simulink model "DDCU_wxt_v02_forA"  (R2014a)
settings: Solver=FixedStepDiscrete  StartTime=0.0  StopTime=50  FixedStep=0.0005  RelTol=1e-3
InitFcn:
  | Veh_Par_wxt
values from neighbouring files (symbols this model uses):
  ag_thr = 0.4*g    (= 3.924)    [Veh_Par_wxt.m]
  B = 2.25    [Veh_Par_wxt.m]
  bra_pre_em = 12    [Veh_Par_wxt.m]
  bra_pre_gz2 = 12/3    (= 4)    [Veh_Par_wxt.m]
  bra_pre_gz34 = 12/3    (= 4)    [Veh_Par_wxt.m]
  bra_pre_yd = 12/2    (= 6)    [Veh_Par_wxt.m]
  brakepre_dem_data = [0 1 2 3 4 5 6 7 8 9 10 11 12]    [Veh_Par_wxt.m]
  brakeTrq_dem_data = [0 218.198 436.396 654.594 872.792 1090.99 1309.188 1527.386 1745.584 1963.782 2181.98 2400.178 2618.376]    [Veh_Par_wxt.m]
  bratrq_max = 4*2618.376    (= 10473.504)    [Veh_Par_wxt.m]
  eff_tran = 0.75    [Veh_Par_wxt.m]
  G = Mass*g    (= 36297)    [Veh_Par_wxt.m]
  kd1 = 1    [Veh_Par_wxt.m]
  kd2 = 1    [Veh_Par_wxt.m]
  kd3 = 1    [Veh_Par_wxt.m]
  ki1 = 1    [Veh_Par_wxt.m]
  ki2 = 1    [Veh_Par_wxt.m]
  ki3 = 1    [Veh_Par_wxt.m]
  kp1 = 1    [Veh_Par_wxt.m]
  kp2 = 1    [Veh_Par_wxt.m]
  kp3 = 1    [Veh_Par_wxt.m]
  L = 3.12    [Veh_Par_wxt.m]
  Radius = 0.20    (= 0.2)    [Veh_Par_wxt.m]
  s_opt_yi_add = 0.05    [Veh_Par_wxt.m]
  s_opt_zhuan_add = 0.05    [Veh_Par_wxt.m]
  spd_map_mot = [0 100 200 300 360 400 500 600 700 800 900]*tras_ratio    [Veh_Par_wxt.m]
  speed_thr_park = 5/3.6/Radius*30/pi    (= 66.3145596216)    [Veh_Par_wxt.m]
  trq_map_mot = [1200 1200 1200 1200 1200 1080 864 720 617 540 480]/tras_ratio    [Veh_Par_wxt.m]
  v_thr1_b = 5    [Veh_Par_wxt.m]
  v_thr2_b = 20    [Veh_Par_wxt.m]
  v_thr_park = 5    [Veh_Par_wxt.m]
undefined symbols (not defined in the file or in its folder): DiscIntNeverNeededParam
libraries: simulink x201, ec5744lib x19
(part 1 of 9)
settings Model: Creator=wxt  LastModifiedBy=wxt
settings OptimizationCC: InlineParams=on  InlineInvariantSignals=on  ExpressionFolding=off  RollThreshold=9  StateBitsets=on  DataBitsets=on  UseTempVars=on  ZeroExternalMemoryAtStartup=off  ZeroInternalMemoryAtStartup=off  EfficientFloat2IntCast=on  OptimizeModelRefInitCode=on  LifeSpan=1
settings DebuggingCC: InheritedTsInSrcMsg=none
settings HardwareCC: ProdLargestAtomicInteger=Long  ProdLargestAtomicFloat=Double  ProdIntDivRoundTo=Zero  ProdEndianess=BigEndian  ProdHWDeviceType=Freescale MPC5500
settings RTWCC: SystemTargetFile=ec5744.tlc  MakeCommand=make_rtw optimized_fixed_point=1  GenerateMakefile=off  TemplateMakefile=ec5744_lcc.tmf  PostCodeGenCommand=ec5744_pst_s2(buildInfo)  Description=Target for EC5744  GenerateReport=on  ProcessScript=ec5744_make_rtw_hook  IncludeHyperlinkInReport=on  LaunchReport=on
settings CodeAppCC: IgnoreCustomStorageClasses=off
settings STFCustomTargetCC: ModelReferenceCompliant=off  ConcurrentExecutionCompliant=off  IncludeMdlTerminateFcn=off  GeneratePreprocessorConditionals=Use local settings  CombineOutputUpdateFcns=on  SuppressErrorStatus=on  ERTCustomFileBanners=on  SupportContinuousTime=off  SupportNonInlinedSFcns=off  MATLABClassNameForMDSCustomization=Simulink.SoftwareTarget.ERTCustomization  GRTInterface=off  SystemTargetFile=ec5744.tlc
settings ERTTargetCC: GenerateSampleERTMain=off  ModelReferenceCompliant=off  IncludeMdlTerminateFcn=off  SuppressErrorStatus=on  GenerateASAP2=on  ERTSrcFileBannerTemplate=ec5744_code_template.cgt  ERTHdrFileBannerTemplate=ec5744_code_template.cgt  ERTDataSrcFileTemplate=ec5744_code_template.cgt  ERTDataHdrFileTemplate=ec5744_code_template.cgt  ERTCustomFileTemplate=ec5744_file_process.tlc

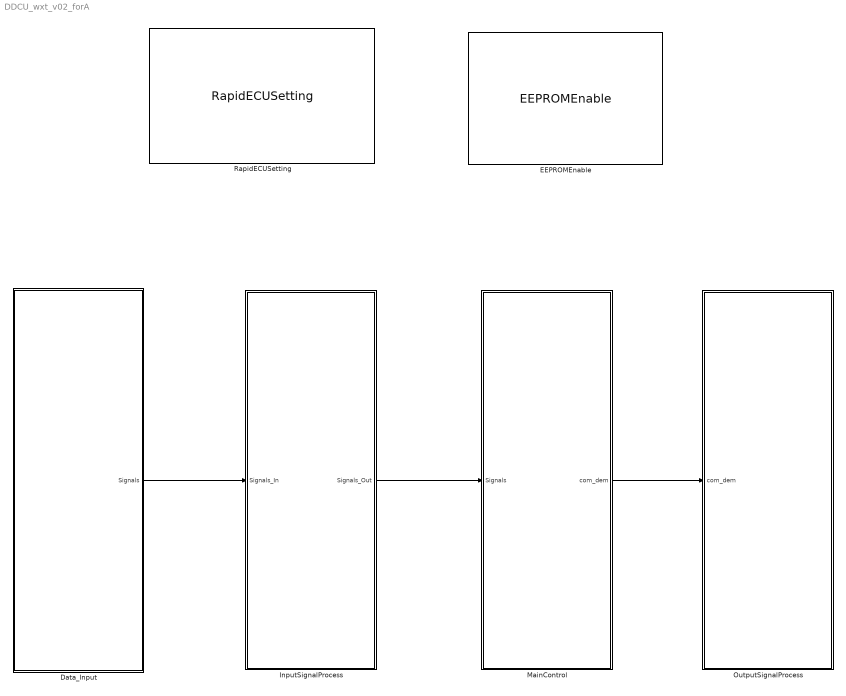
== system DDCU_wxt_v02_forA ==
  Data_Input : Subsystem
  EEPROMEnable : ec5744lib/RapidECU_U3/09MemoryManagement/EEPROMEnable  eepromenable=on
  InputSignalProcess : Subsystem
  MainControl : Subsystem
  OutputSignalProcess : Subsystem
  RapidECUSetting : ec5744lib/RapidECU_U3/RapidECUSetting
      link override CAN: apdf=4  bpdf=4  cpdf=4  acmt=Extended(29-bit ID)  bcmt=Extended(29-bit ID)
      link override LIN: abrt=19200
  wires:
  Data_Input/1(Signals) -> InputSignalProcess/1(Signals_In)
  InputSignalProcess/1(Signals_Out) -> MainControl/1(Signals)
  MainControl/1(com_dem) -> OutputSignalProcess/1(com_dem)

== system DDCU_wxt_v02_forA/Data_Input ==
  Battery : Subsystem
  BraSystem : Subsystem
  Bus Creator : BusCreator  Inputs=6
  DriveMotor : Subsystem
  ESC2VCU : Subsystem
  Ground : Ground
  Ground1 : Ground
  Ground2 : Ground
  HCU2VCU : Subsystem
  IMU : Subsystem
  MCU2VCU : Subsystem
  Subsystem : Subsystem
  Suspension : Subsystem
  YaoKong : Subsystem
  Signals : Outport
  wires:
  DriveMotor/1(DriveMotor) -> Bus Creator/2
  BraSystem/1(BraPre) -> Bus Creator/3
  YaoKong/1(YaoKong_dem) -> Bus Creator/1
  IMU/1(IMU) -> Bus Creator/4
  Suspension/1(Center_of_Mass) -> Bus Creator/5
  Bus Creator/1 -> Signals/1
  Battery/1(Bat) -> Bus Creator/6
  Ground/1 -> Suspension/1(location_center)
  Ground2/1 -> Battery/2(pwr_chg_bat)
  Ground1/1 -> Battery/1(pwr_dis_bat)
  HCU2VCU/5(Turn_Out) -> YaoKong/3(steer_dem)
  HCU2VCU/6(AccBra_Out) -> YaoKong/2(acc_dem)
  HCU2VCU/7(Mode2_Out) -> Subsystem/1(Mode2_Out)
  HCU2VCU/8(Mode1_Out) -> Subsystem/2(Mode1_Out)
  Subsystem/1(mode_dem) -> YaoKong/1(mode_dem)
  MCU2VCU/2(M1Speed_Out) -> DriveMotor/1(speed_act_lf)
  MCU2VCU/7(M1Torque_Out) -> DriveMotor/2(trq_act_lf)
  MCU2VCU/8(M1FaultGrade_Out) -> DriveMotor/5(guzhang_lf)
  MCU2VCU/10(M1TqLimit_Out) -> DriveMotor/3(trqlimU_dig_lf)
  MCU2VCU/14(M3Speed_Out) -> DriveMotor/6(speed_act_lr)
  MCU2VCU/19(M3Torque_Out) -> DriveMotor/7(trq_act_lr)
  MCU2VCU/21(M3FaultGrade_Out) -> DriveMotor/10(guzhang_lr)
  MCU2VCU/22(M3TqLimit_Out) -> DriveMotor/8(trqlimU_dig_lr)
  MCU2VCU/25(M2Torque_Out) -> DriveMotor/12(trq_act_rf)
  MCU2VCU/27(M2Speed_Out) -> DriveMotor/11(speed_act_rf)
  MCU2VCU/33(M2FaultGrade_Out) -> DriveMotor/15(guzhang_rf)
  MCU2VCU/34(M2TqLimit_Out) -> DriveMotor/13(trqlimU_dig_rf)
  MCU2VCU/38(M4Speed_Out) -> DriveMotor/16(speed_act_rr)
  MCU2VCU/43(M4Torque_Out) -> DriveMotor/17(trq_act_rr)
  MCU2VCU/45(M4FaultGrade_Out) -> DriveMotor/20(guzhang_rr)
  MCU2VCU/46(M4TqLimit_Out) -> DriveMotor/18(trqlimU_dig_rr)
  ESC2VCU/11(VESC_BrkPLe_MPa_Out) -> BraSystem/1(BraPre_act_l)
  ESC2VCU/10(VESC_BrkPRi_MPa_Out) -> BraSystem/2(BraPre_act_r)

== system DDCU_wxt_v02_forA/InputSignalProcess ==
  note: 注：所有的单位转换都发生在此模块
      | 速度 km/h
      | 角速度 rpm
      | 加速度信号0-100
      | 制动信号0-100
      | 向左为正
  Signals_In : Inport
  Signals_Out : Outport
  wires:
  Signals_In/1 -> Signals_Out/1

== system DDCU_wxt_v02_forA/MainControl ==
  Signals : Inport
  mode_control : Subsystem
  mode_switch : Subsystem
  com_dem : Outport
  wires:
  Signals/1 -> mode_control/2(Signals), mode_switch/1(Signals)
  mode_switch/1(mode_dem_out) -> mode_control/1(mode_dem_out)
  mode_control/1(com_dem) -> com_dem/1

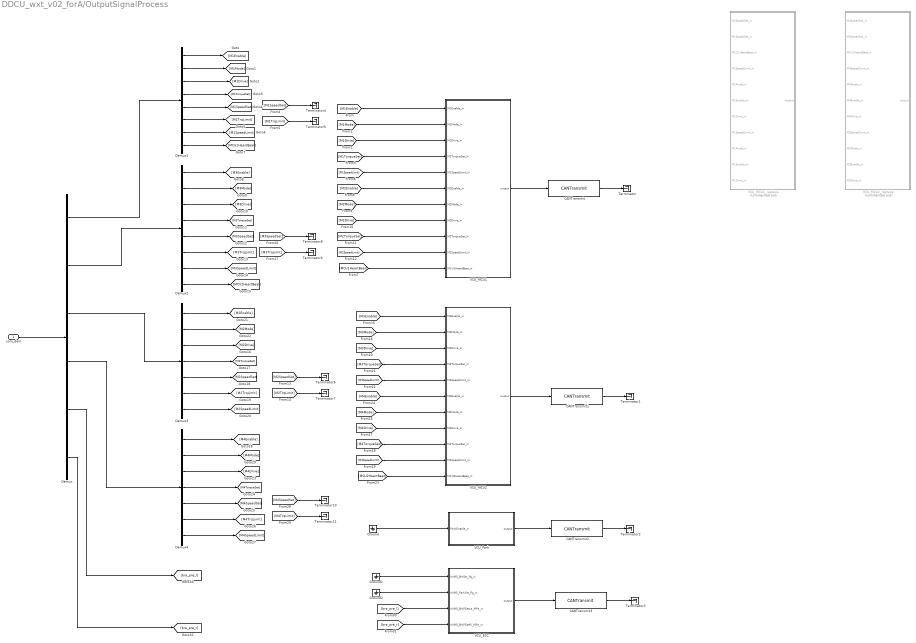
== system DDCU_wxt_v02_forA/OutputSignalProcess ==
  com_dem : Inport
  CANTransmit : ec5744lib/RapidECU_U3/04CANCommunication/CANTransmit  canmodule=0  canbuffer=8  canmessageid=hex2dec('0C01F001')  canmessagetype=Extended(29-bit ID)  datalength=8  sampletime=-1
  CANTransmit1 : ec5744lib/RapidECU_U3/04CANCommunication/CANTransmit  canmodule=0  canbuffer=9  canmessageid=hex2dec('0C01F002')  canmessagetype=Extended(29-bit ID)  datalength=8  sampletime=-1
  CANTransmit2 : ec5744lib/RapidECU_U3/04CANCommunication/CANTransmit  canmodule=1  canbuffer=10  canmessageid=hex2dec('804623A')  canmessagetype=Extended(29-bit ID)  datalength=8  sampletime=-1
  CANTransmit3 : ec5744lib/RapidECU_U3/04CANCommunication/CANTransmit  canmodule=1  canbuffer=11  canmessageid=hex2dec('0CF6EAF0')  canmessagetype=Extended(29-bit ID)  datalength=8  sampletime=-1
  Demux : Demux  Outputs=6
  Demux1 : Demux  Outputs=8
  Demux2 : Demux  Outputs=8
  Demux3 : Demux  Outputs=7
  Demux4 : Demux  Outputs=7
  Ground : Ground
  Ground1 : Ground
  Ground2 : Ground
  Terminator{,1..11} (12 alike) : Terminator
  VCU_ESC : Subsystem
  VCU_MCU1 : Subsystem
  VCU_MCU1_replace : Subsystem  Commented=on
  VCU_MCU2 : Subsystem
  VCU_MCU2_replace : Subsystem  Commented=on
  VCU_Park : Subsystem
  wires:
  com_dem/1 -> Demux/1
  Demux/1 -> Demux1/1
  Demux/2 -> Demux2/1
  Demux/3 -> Demux3/1
  Demux/4 -> Demux4/1
  CANTransmit/1 -> Terminator/1
  CANTransmit1/1 -> Terminator1/1
  VCU_MCU2/1(output) -> CANTransmit1/1
  CANTransmit2/1 -> Terminator2/1
  VCU_Park/1(output) -> CANTransmit2/1
  CANTransmit3/1 -> Terminator3/1
  VCU_ESC/1(output) -> CANTransmit3/1
  Demux1/3 -> [M1Drive]
  Demux1/4 -> [M1TorqueSet]
  Demux1/2 -> [M1Mode]
  Demux1/5 -> [M1SpeedSet]
  Demux1/6 -> [M1TrqLimit]
  Demux1/1 -> [M1Enable]
  Demux1/7 -> [M1SpeedLimit]
  Demux1/8 -> [MCU1HeartBeat]
  Demux2/7 -> [M3SpeedLimit]
  Demux2/6 -> [M3TrqLimit]
  Demux2/1 -> [M3Enable]
  Demux2/8 -> [MCU2HeartBeat]
  Demux2/5 -> [M3SpeedSet]
  Demux2/2 -> [M3Mode]
  Demux2/4 -> [M3TorqueSet]
  Demux2/3 -> [M3Drive]
  Demux3/1 -> [M2Enable]
  Demux3/6 -> [M2TrqLimit]
  Demux3/7 -> [M2SpeedLimit]
  Demux3/5 -> [M2SpeedSet]
  Demux3/4 -> [M2TorqueSet]
  Demux3/2 -> [M2Mode]
  Demux3/3 -> [M2Drive]
  Demux4/1 -> [M4Enable]
  Demux4/2 -> [M4Mode]
  Demux4/3 -> [M4Drive]
  Demux4/4 -> [M4TorqueSet]
  Demux4/5 -> [M4SpeedSet]
  Demux4/6 -> [M4TrqLimit]
  Demux4/7 -> [M4SpeedLimit]
  [M1Enable] -> VCU_MCU1/1(M1Enable_in)
  [M1Mode] -> VCU_MCU1/2(M1Mode_in)
  [M1Drive] -> VCU_MCU1/3(M1Drive_in)
  [M1TorqueSet] -> VCU_MCU1/4(M1TorqueSet_in)
  [M1SpeedSet] -> Terminator4/1
  [M1TrqLimit] -> Terminator5/1
  [M1SpeedLimit] -> VCU_MCU1/5(M1SpeedLimit_in)
  [MCU1HeartBeat] -> VCU_MCU1/11(MCU1HeartBeat_in)
  [M2TorqueSet] -> VCU_MCU1/9(M2TorqueSet_in)
  [M2SpeedLimit] -> VCU_MCU1/10(M2SpeedLimit_in)
  [M2Enable] -> VCU_MCU1/6(M2Enable_in)
  [M2Drive] -> VCU_MCU1/8(M2Drive_in)
  [M2Mode] -> VCU_MCU1/7(M2Mode_in)
  [M2SpeedSet] -> Terminator6/1
  [M2TrqLimit] -> Terminator7/1
  [MCU2HeartBeat] -> VCU_MCU2/11(MCU2HeartBeat_in)
  [M4TorqueSet] -> VCU_MCU2/9(M4TorqueSet_in)
  [M3TorqueSet] -> VCU_MCU2/4(M3TorqueSet_in)
  [M3SpeedLimit] -> VCU_MCU2/5(M3SpeedLimit_in)
  [M4SpeedLimit] -> VCU_MCU2/10(M4SpeedLimit_in)
  [M3Enable] -> VCU_MCU2/1(M3Enable_in)
  [M4Enable] -> VCU_MCU2/6(M4Enable_in)
  [M3Mode] -> VCU_MCU2/2(M3Mode_in)
  [M4Drive] -> VCU_MCU2/8(M4Drive_in)
  [M3Drive] -> VCU_MCU2/3(M3Drive_in)
  [M4Mode] -> VCU_MCU2/7(M4Mode_in)
  [M3SpeedSet] -> Terminator8/1
  [M3TrqLimit] -> Terminator9/1
  [M4SpeedSet] -> Terminator10/1
  [M4TrqLimit] -> Terminator11/1
  Demux/5 -> [bra_pre_l]
  Demux/6 -> [bra_pre_r]
  [bra_pre_l] -> VCU_ESC/3(VVMS_BrkPSetLe_MPa_in)
  [bra_pre_r] -> VCU_ESC/4(VVMS_BrkPSetRi_MPa_in)
  Ground/1 -> VCU_Park/1(ParkEnable_in)
  Ground1/1 -> VCU_ESC/1(VVMS_BrkSts_flg_in)
  Ground2/1 -> VCU_ESC/2(VVMS_ParkSts_flg_in)
  VCU_MCU1/1(output) -> CANTransmit/1

== system DDCU_wxt_v02_forA/Data_Input/Battery ==
  pwr_dis_bat : Inport
  pwr_chg_bat : Inport  Port=2
  Bus Creator : BusCreator  Inputs=2
  Bat : Outport
  wires:
  pwr_dis_bat/1 -> Bus Creator/1  "pwr_dis_bat"
  Bus Creator/1 -> Bat/1  "Bat"
  pwr_chg_bat/1 -> Bus Creator/2  "pwr_chg_bat"

== system DDCU_wxt_v02_forA/Data_Input/BraSystem ==
  BraPre_act_l : Inport
  BraPre_act_r : Inport  Port=2
  Bus Creator : BusCreator  Inputs=2
  BraPre : Outport
  wires:
  BraPre_act_l/1 -> Bus Creator/1  "BraPre_act"
  Bus Creator/1 -> BraPre/1  "BraPre"
  BraPre_act_r/1 -> Bus Creator/2  "BraPre_act_r"

== system DDCU_wxt_v02_forA/Data_Input/DriveMotor ==
  speed_act_lf : Inport
  trq_act_lf : Inport  Port=2
  trqlimU_dig_lf : Inport  Port=3
  trqlimL_dig_lf : Inport  Port=4
  guzhang_lf : Inport  Port=5
  speed_act_lr : Inport  Port=6
  trq_act_lr : Inport  Port=7
  trqlimU_dig_lr : Inport  Port=8
  trqlimL_dig_lr : Inport  Port=9
  guzhang_lr : Inport  Port=10
  speed_act_rf : Inport  Port=11
  trq_act_rf : Inport  Port=12
  trqlimU_dig_rf : Inport  Port=13
  trqlimL_dig_rf : Inport  Port=14
  guzhang_rf : Inport  Port=15
  speed_act_rr : Inport  Port=16
  trq_act_rr : Inport  Port=17
  trqlimU_dig_rr : Inport  Port=18
  trqlimL_dig_rr : Inport  Port=19
  guzhang_rr : Inport  Port=20
  Bus Creator : BusCreator  Inputs=20
  DriveMotor : Outport
  wires:
  Bus Creator/1 -> DriveMotor/1  "DriveMotor"
  trqlimL_dig_lr/1 -> Bus Creator/9  "trqlimL_dig_lr"
  trq_act_lf/1 -> Bus Creator/2  "trq_act_lf"
  trq_act_lr/1 -> Bus Creator/7  "trq_act_lr"
  trqlimL_dig_lf/1 -> Bus Creator/4  "trqlimL_dig_lf"
  trqlimU_dig_lf/1 -> Bus Creator/3  "trqlimU_dig_lf"
  trqlimU_dig_lr/1 -> Bus Creator/8  "trqlimU_dig_lr"
  speed_act_lf/1 -> Bus Creator/1  "speed_act_lf"
  speed_act_lr/1 -> Bus Creator/6  "speed_act_lr"
  guzhang_rf/1 -> Bus Creator/15  "guzhang_rf"
  guzhang_lf/1 -> Bus Creator/5  "guzhang_lf"
  guzhang_lr/1 -> Bus Creator/10  "guzhang_lr"
  speed_act_rf/1 -> Bus Creator/11  "speed_act_rf"
  guzhang_rr/1 -> Bus Creator/20  "guzhang_rr"
  trq_act_rf/1 -> Bus Creator/12  "trq_act_rf"
  speed_act_rr/1 -> Bus Creator/16  "speed_act_rr"
  trqlimL_dig_rf/1 -> Bus Creator/14  "trqlimL_dig_rf"
  trq_act_rr/1 -> Bus Creator/17  "trq_act_rr"
  trqlimL_dig_rr/1 -> Bus Creator/19  "trqlimL_dig_rr"
  trqlimU_dig_rf/1 -> Bus Creator/13  "trqlimU_dig_rf"
  trqlimU_dig_rr/1 -> Bus Creator/18  "trqlimU_dig_rr"

== system DDCU_wxt_v02_forA/Data_Input/ESC2VCU ==
  CANReceive : ec5744lib/RapidECU_U3/04CANCommunication/CANReceive  canmodule=1  canbuffer=18  canmessageid=hex2dec('D022466')  canmessagetype=Extended(29-bit ID)  datalength=8  sampletime=-1
  CANReceive1 : ec5744lib/RapidECU_U3/04CANCommunication/CANReceive  canmodule=1  canbuffer=19  canmessageid=hex2dec('1002247A')  canmessagetype=Extended(29-bit ID)  datalength=8  sampletime=-1
  CANReceive2 : ec5744lib/RapidECU_U3/04CANCommunication/CANReceive  canmodule=1  canbuffer=20  canmessageid=hex2dec('0CF6F0EA')  canmessagetype=Extended(29-bit ID)  datalength=8  sampletime=-1
  ESC_VCU : Subsystem
  Park1_VCU : Subsystem
  Park2_VCU : Subsystem
  Terminator{,1..8} (9 alike) : Terminator
  ParkZiJian_Out : Outport
  ParkState_Out : Outport  Port=2
  VESC_BrkPMa_MPa_Out : Outport  Port=3
  VESC_BrkPSetRi_MPa_Out : Outport  Port=4
  VESC_BrkPSetLe_MPa_Out : Outport  Port=5
  VESC_BrkFlt_enum_Out : Outport  Port=6
  VESC_HotSts_flg_Out : Outport  Port=7
  VESC_BrkReq_flg_Out : Outport  Port=8
  VESC_ParkReq_flg_Out : Outport  Port=9
  VESC_BrkPRi_MPa_Out : Outport  Port=10
  VESC_BrkPLe_MPa_Out : Outport  Port=11
  wires:
  CANReceive/4 -> Park1_VCU/1(input)
  CANReceive/5 -> Terminator2/1
  CANReceive/3 -> Terminator1/1
  CANReceive/2 -> Terminator/1
  CANReceive1/4 -> Park2_VCU/1(input)
  CANReceive1/2 -> Terminator3/1
  CANReceive1/3 -> Terminator4/1
  CANReceive1/5 -> Terminator5/1
  CANReceive2/4 -> ESC_VCU/1(input)
  CANReceive2/5 -> Terminator8/1
  CANReceive2/2 -> Terminator6/1
  CANReceive2/3 -> Terminator7/1
  Park1_VCU/1(ParkZiJian_Out) -> ParkZiJian_Out/1
  Park2_VCU/1(ParkState_Out) -> ParkState_Out/1
  ESC_VCU/1(VESC_BrkPMa_MPa_Out) -> VESC_BrkPMa_MPa_Out/1
  ESC_VCU/2(VESC_BrkPSetRi_MPa_Out) -> VESC_BrkPSetRi_MPa_Out/1
  ESC_VCU/3(VESC_BrkPSetLe_MPa_Out) -> VESC_BrkPSetLe_MPa_Out/1
  ESC_VCU/4(VESC_BrkFlt_enum_Out) -> VESC_BrkFlt_enum_Out/1
  ESC_VCU/5(VESC_HotSts_flg_Out) -> VESC_HotSts_flg_Out/1
  ESC_VCU/6(VESC_BrkReq_flg_Out) -> VESC_BrkReq_flg_Out/1
  ESC_VCU/7(VESC_ParkReq_flg_Out) -> VESC_ParkReq_flg_Out/1
  ESC_VCU/8(VESC_BrkPRi_MPa_Out) -> VESC_BrkPRi_MPa_Out/1
  ESC_VCU/9(VESC_BrkPLe_MPa_Out) -> VESC_BrkPLe_MPa_Out/1
  CANReceive/1 -> Park1_VCU/Trigger
  CANReceive1/1 -> Park2_VCU/Trigger
  CANReceive2/1 -> ESC_VCU/Trigger

== system DDCU_wxt_v02_forA/Data_Input/HCU2VCU ==
  CANReceive : ec5744lib/RapidECU_U3/04CANCommunication/CANReceive  canmodule=0  canbuffer=0  canmessageid=hex2dec('1502C23A')  canmessagetype=Extended(29-bit ID)  datalength=8  sampletime=-1
  CANReceive1 : ec5744lib/RapidECU_U3/04CANCommunication/CANReceive  canmodule=0  canbuffer=1  canmessageid=hex2dec('902C23A')  canmessagetype=Extended(29-bit ID)  datalength=8  sampletime=-1
  HCU1_VCU : Subsystem
  HCU2_VCU : Subsystem
  Terminator{,1..5} (6 alike) : Terminator
  VehEnvironment_Out : Outport
  KeyState_Out : Outport  Port=2
  VehFault_Out : Outport  Port=3
  HCUState_Out : Outport  Port=4
  Turn_Out : Outport  Port=5
  AccBra_Out : Outport  Port=6
  Mode2_Out : Outport  Port=7
  Mode1_Out : Outport  Port=8
  wires:
  CANReceive/1 -> HCU1_VCU/Trigger
  CANReceive/2 -> Terminator/1
  CANReceive/3 -> Terminator1/1
  CANReceive/4 -> HCU1_VCU/1(input)
  CANReceive/5 -> Terminator2/1
  CANReceive1/4 -> HCU2_VCU/1(input)
  CANReceive1/5 -> Terminator5/1
  CANReceive1/2 -> Terminator3/1
  CANReceive1/3 -> Terminator4/1
  HCU1_VCU/1(VehEnvironment_Out) -> VehEnvironment_Out/1
  HCU1_VCU/2(KeyState_Out) -> KeyState_Out/1
  HCU1_VCU/3(VehFault_Out) -> VehFault_Out/1
  HCU1_VCU/4(HCUState_Out) -> HCUState_Out/1
  HCU2_VCU/1(Turn_Out) -> Turn_Out/1
  HCU2_VCU/2(AccBra_Out) -> AccBra_Out/1
  HCU2_VCU/3(Mode2_Out) -> Mode2_Out/1
  HCU2_VCU/4(Mode1_Out) -> Mode1_Out/1
  CANReceive1/1 -> HCU2_VCU/Trigger

== system DDCU_wxt_v02_forA/Data_Input/IMU ==
  v_act : Inport
  dis_east : Inport  Port=2
  dis_north : Inport  Port=3
  dis_sky : Inport  Port=4
  hangxiangangle : Inport  Port=5
  fuyangangle : Inport  Port=6
  henggunangle : Inport  Port=7
  acc_x : Inport  Port=8
  acc_y : Inport  Port=9
  acc_z : Inport  Port=10
  jiaosudu_x : Inport  Port=11
  jiaosudu_y : Inport  Port=12
  jiaosudu_z : Inport  Port=13
  Bus Creator : BusCreator  Inputs=13
  IMU : Outport
  wires:
  Bus Creator/1 -> IMU/1  "IMU"
  dis_east/1 -> Bus Creator/2  "dis_east"
  hangxiangangle/1 -> Bus Creator/5  "hangxiangangle"
  dis_north/1 -> Bus Creator/3  "dis_north"
  dis_sky/1 -> Bus Creator/4  "dis_sky"
  fuyangangle/1 -> Bus Creator/6  "fuyangangle"
  acc_y/1 -> Bus Creator/9  "acc_y"
  henggunangle/1 -> Bus Creator/7  "henggunangle"
  acc_x/1 -> Bus Creator/8  "acc_x"
  acc_z/1 -> Bus Creator/10  "acc_z"
  jiaosudu_z/1 -> Bus Creator/13  "jiaosudu_z"
  jiaosudu_x/1 -> Bus Creator/11  "jiaosudu_x"
  jiaosudu_y/1 -> Bus Creator/12  "jiaosudu_y"
  v_act/1 -> Bus Creator/1  "v_act"

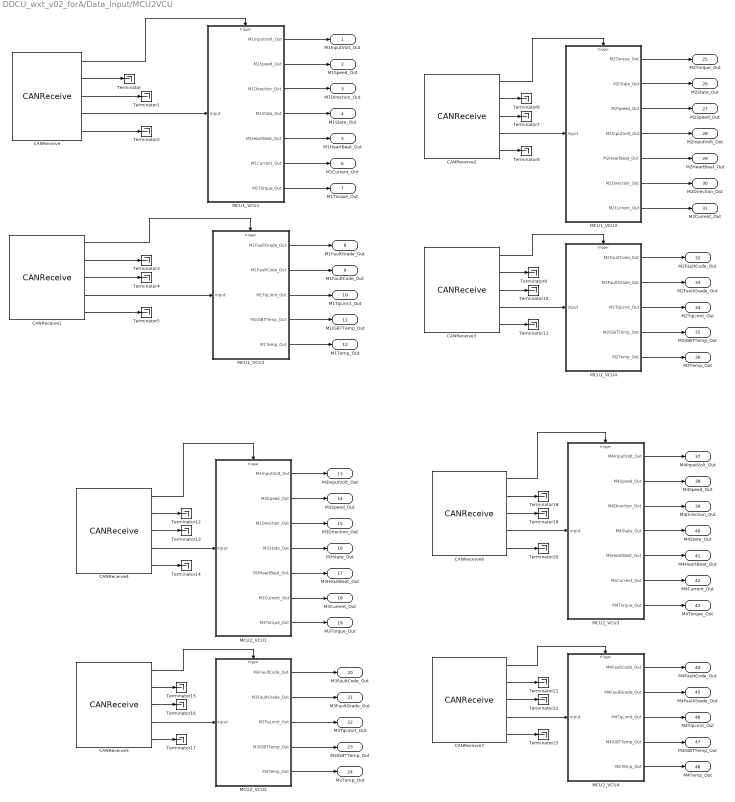
== system DDCU_wxt_v02_forA/Data_Input/MCU2VCU ==
  CANReceive : ec5744lib/RapidECU_U3/04CANCommunication/CANReceive  canmodule=0  canbuffer=2  canmessageid=hex2dec('0C0101F0')  canmessagetype=Extended(29-bit ID)  datalength=8  sampletime=-1
  CANReceive1 : ec5744lib/RapidECU_U3/04CANCommunication/CANReceive  canmodule=0  canbuffer=3  canmessageid=hex2dec('0C0201F0')  canmessagetype=Extended(29-bit ID)  datalength=8  sampletime=-1
  CANReceive2 : ec5744lib/RapidECU_U3/04CANCommunication/CANReceive  canmodule=0  canbuffer=4  canmessageid=hex2dec('0C0301F0')  canmessagetype=Extended(29-bit ID)  datalength=8  sampletime=-1
  CANReceive3 : ec5744lib/RapidECU_U3/04CANCommunication/CANReceive  canmodule=0  canbuffer=5  canmessageid=hex2dec('0C0401F0')  canmessagetype=Extended(29-bit ID)  datalength=8  sampletime=-1
  CANReceive4 : ec5744lib/RapidECU_U3/04CANCommunication/CANReceive  canmodule=0  canbuffer=6  canmessageid=hex2dec('0C0102F0')  canmessagetype=Extended(29-bit ID)  datalength=8  sampletime=-1
  CANReceive5 : ec5744lib/RapidECU_U3/04CANCommunication/CANReceive  canmodule=0  canbuffer=7  canmessageid=hex2dec('0C0202F0')  canmessagetype=Extended(29-bit ID)  datalength=8  sampletime=-1
  CANReceive6 : ec5744lib/RapidECU_U3/04CANCommunication/CANReceive  canmodule=0  canbuffer=16  canmessageid=hex2dec('0C0302F0')  canmessagetype=Extended(29-bit ID)  datalength=8  sampletime=-1
  CANReceive7 : ec5744lib/RapidECU_U3/04CANCommunication/CANReceive  canmodule=0  canbuffer=17  canmessageid=hex2dec('0C0402F0')  canmessagetype=Extended(29-bit ID)  datalength=8  sampletime=-1
  MCU1_VCU1 : Subsystem
  MCU1_VCU2 : Subsystem
  MCU1_VCU3 : Subsystem
  MCU1_VCU4 : Subsystem
  MCU2_VCU1 : Subsystem
  MCU2_VCU2 : Subsystem
  MCU2_VCU3 : Subsystem
  MCU2_VCU4 : Subsystem
  Terminator{,1..23} (24 alike) : Terminator
  M1InputVolt_Out : Outport
  M1Speed_Out : Outport  Port=2
  M1Direction_Out : Outport  Port=3
  M1State_Out : Outport  Port=4
  M1HeartBeat_Out : Outport  Port=5
  M1Current_Out : Outport  Port=6
  M1Torque_Out : Outport  Port=7
  M1FaultGrade_Out : Outport  Port=8
  M1FaultCode_Out : Outport  Port=9
  M1TqLimit_Out : Outport  Port=10
  M1IGBTTemp_Out : Outport  Port=11
  M1Temp_Out : Outport  Port=12
  M3InputVolt_Out : Outport  Port=13
  M3Speed_Out : Outport  Port=14
  M3Direction_Out : Outport  Port=15
  M3State_Out : Outport  Port=16
  M3HeartBeat_Out : Outport  Port=17
  M3Current_Out : Outport  Port=18
  M3Torque_Out : Outport  Port=19
  M3FaultCode_Out : Outport  Port=20
  M3FaultGrade_Out : Outport  Port=21
  M3TqLimit_Out : Outport  Port=22
  M3IGBTTemp_Out : Outport  Port=23
  M3Temp_Out : Outport  Port=24
  M2Torque_Out : Outport  Port=25
  M2State_Out : Outport  Port=26
  M2Speed_Out : Outport  Port=27
  M2InputVolt_Out : Outport  Port=28
  M2HeartBeat_Out : Outport  Port=29
  M2Direction_Out : Outport  Port=30
  M2Current_Out : Outport  Port=31
  M2FaultCode_Out : Outport  Port=32
  M2FaultGrade_Out : Outport  Port=33
  M2TqLimit_Out : Outport  Port=34
  M2IGBTTemp_Out : Outport  Port=35
  M2Temp_Out : Outport  Port=36
  M4InputVolt_Out : Outport  Port=37
  M4Speed_Out : Outport  Port=38
  M4Direction_Out : Outport  Port=39
  M4State_Out : Outport  Port=40
  M4HeartBeat_Out : Outport  Port=41
  M4Current_Out : Outport  Port=42
  M4Torque_Out : Outport  Port=43
  M4FaultCode_Out : Outport  Port=44
  M4FaultGrade_Out : Outport  Port=45
  M4TqLimit_Out : Outport  Port=46
  M4IGBTTemp_Out : Outport  Port=47
  M4Temp_Out : Outport  Port=48
  wires:
  CANReceive/4 -> MCU1_VCU1/1(input)
  CANReceive/2 -> Terminator/1
  CANReceive/3 -> Terminator1/1
  CANReceive/5 -> Terminator2/1
  CANReceive1/4 -> MCU1_VCU2/1(input)
  CANReceive1/2 -> Terminator3/1
  CANReceive1/3 -> Terminator4/1
  CANReceive1/5 -> Terminator5/1
  CANReceive2/4 -> MCU1_VCU3/1(input)
  CANReceive3/4 -> MCU1_VCU4/1(input)
  CANReceive2/5 -> Terminator8/1
  CANReceive2/2 -> Terminator6/1
  CANReceive2/3 -> Terminator7/1
  CANReceive3/3 -> Terminator10/1
  CANReceive3/5 -> Terminator11/1
  CANReceive3/2 -> Terminator9/1
  CANReceive4/4 -> MCU2_VCU1/1(input)
  CANReceive4/2 -> Terminator12/1
  CANReceive4/3 -> Terminator13/1
  CANReceive4/5 -> Terminator14/1
  CANReceive5/4 -> MCU2_VCU2/1(input)
  CANReceive5/2 -> Terminator15/1
  CANReceive5/3 -> Terminator16/1
  CANReceive5/5 -> Terminator17/1
  CANReceive6/4 -> MCU2_VCU3/1(input)
  CANReceive6/2 -> Terminator18/1
  CANReceive6/3 -> Terminator19/1
  CANReceive6/5 -> Terminator20/1
  CANReceive7/4 -> MCU2_VCU4/1(input)
  CANReceive7/2 -> Terminator21/1
  CANReceive7/3 -> Terminator22/1
  CANReceive7/5 -> Terminator23/1
  MCU1_VCU1/7(M1Torque_Out) -> M1Torque_Out/1
  MCU1_VCU1/6(M1Current_Out) -> M1Current_Out/1
  MCU1_VCU1/5(M1HeartBeat_Out) -> M1HeartBeat_Out/1
  MCU1_VCU1/4(M1State_Out) -> M1State_Out/1
  MCU1_VCU1/3(M1Direction_Out) -> M1Direction_Out/1
  MCU1_VCU1/2(M1Speed_Out) -> M1Speed_Out/1
  MCU1_VCU1/1(M1InputVolt_Out) -> M1InputVolt_Out/1
  MCU1_VCU2/5(M1Temp_Out) -> M1Temp_Out/1
  MCU1_VCU2/4(M1IGBTTemp_Out) -> M1IGBTTemp_Out/1
  MCU1_VCU2/3(M1TqLimit_Out) -> M1TqLimit_Out/1
  MCU1_VCU2/2(M1FaultCode_Out) -> M1FaultCode_Out/1
  MCU1_VCU2/1(M1FaultGrade_Out) -> M1FaultGrade_Out/1
  MCU2_VCU1/1(M3InputVolt_Out) -> M3InputVolt_Out/1
  MCU2_VCU1/2(M3Speed_Out) -> M3Speed_Out/1
  MCU2_VCU1/3(M3Direction_Out) -> M3Direction_Out/1
  MCU2_VCU1/4(M3State_Out) -> M3State_Out/1
  MCU2_VCU1/5(M3HeartBeat_Out) -> M3HeartBeat_Out/1
  MCU2_VCU1/6(M3Current_Out) -> M3Current_Out/1
  MCU2_VCU1/7(M3Torque_Out) -> M3Torque_Out/1
  MCU2_VCU2/1(M3FaultCode_Out) -> M3FaultCode_Out/1
  MCU2_VCU2/2(M3FaultGrade_Out) -> M3FaultGrade_Out/1
  MCU2_VCU2/3(M3TqLimit_Out) -> M3TqLimit_Out/1
  MCU2_VCU2/4(M3IGBTTemp_Out) -> M3IGBTTemp_Out/1
  MCU2_VCU2/5(M3Temp_Out) -> M3Temp_Out/1
  MCU1_VCU3/1(M2Torque_Out) -> M2Torque_Out/1
  MCU1_VCU3/2(M2State_Out) -> M2State_Out/1
  MCU1_VCU3/3(M2Speed_Out) -> M2Speed_Out/1
  MCU1_VCU3/4(M2InputVolt_Out) -> M2InputVolt_Out/1
  MCU1_VCU3/5(M2HeartBeat_Out) -> M2HeartBeat_Out/1
  MCU1_VCU3/6(M2Direction_Out) -> M2Direction_Out/1
  MCU1_VCU3/7(M2Current_Out) -> M2Current_Out/1
  MCU1_VCU4/1(M2FaultCode_Out) -> M2FaultCode_Out/1
  MCU1_VCU4/2(M2FaultGrade_Out) -> M2FaultGrade_Out/1
  MCU1_VCU4/3(M2TqLimit_Out) -> M2TqLimit_Out/1
  MCU1_VCU4/4(M2IGBTTemp_Out) -> M2IGBTTemp_Out/1
  MCU1_VCU4/5(M2Temp_Out) -> M2Temp_Out/1
  MCU2_VCU3/1(M4InputVolt_Out) -> M4InputVolt_Out/1
  MCU2_VCU3/2(M4Speed_Out) -> M4Speed_Out/1
  MCU2_VCU3/3(M4Direction_Out) -> M4Direction_Out/1
  MCU2_VCU3/4(M4State_Out) -> M4State_Out/1
  MCU2_VCU3/5(M4HeartBeat_Out) -> M4HeartBeat_Out/1
  MCU2_VCU3/6(M4Current_Out) -> M4Current_Out/1
  MCU2_VCU3/7(M4Torque_Out) -> M4Torque_Out/1
  MCU2_VCU4/1(M4FaultCode_Out) -> M4FaultCode_Out/1
  MCU2_VCU4/2(M4FaultGrade_Out) -> M4FaultGrade_Out/1
  MCU2_VCU4/3(M4TqLimit_Out) -> M4TqLimit_Out/1
  MCU2_VCU4/4(M4IGBTTemp_Out) -> M4IGBTTemp_Out/1
  MCU2_VCU4/5(M4Temp_Out) -> M4Temp_Out/1
  CANReceive/1 -> MCU1_VCU1/Trigger
  CANReceive1/1 -> MCU1_VCU2/Trigger
  CANReceive2/1 -> MCU1_VCU3/Trigger
  CANReceive3/1 -> MCU1_VCU4/Trigger
  CANReceive4/1 -> MCU2_VCU1/Trigger
  CANReceive5/1 -> MCU2_VCU2/Trigger
  CANReceive6/1 -> MCU2_VCU3/Trigger
  CANReceive7/1 -> MCU2_VCU4/Trigger

== system DDCU_wxt_v02_forA/Data_Input/Subsystem ==
  Mode2_Out : Inport
  Mode1_Out : Inport  Port=2
  MATLAB Function : MATLAB Function  TreatAsAtomicUnit=on
  mode_dem : Outport
  wires:
  Mode1_Out/1 -> MATLAB Function/1(Mode1_Out)
  Mode2_Out/1 -> MATLAB Function/2(Mode2_Out)
  MATLAB Function/1(mode_dem) -> mode_dem/1

== system DDCU_wxt_v02_forA/Data_Input/Suspension ==
  location_center : Inport
  Bus Creator : BusCreator  Inputs=1
  Center_of_Mass : Outport
  wires:
  Bus Creator/1 -> Center_of_Mass/1  "Center_of_Mass"
  location_center/1 -> Bus Creator/1  "location_center"

== system DDCU_wxt_v02_forA/Data_Input/YaoKong ==
  note: 上坡辅助系统(Hill-start Assist Control，HAC)
  mode_dem : Inport
  acc_dem : Inport  Port=2
  steer_dem : Inport  Port=3
  brake_dem : Inport  Port=4
  brake_emerg : Inport  Port=5
  HAC : Inport  Port=6
  Bus Creator : BusCreator  Inputs=6
  YaoKong_dem : Outport
  wires:
  steer_dem/1 -> Bus Creator/3  "steer_dem"
  acc_dem/1 -> Bus Creator/2  "acc_dem"
  brake_dem/1 -> Bus Creator/4  "brake_dem"
  mode_dem/1 -> Bus Creator/1  "mode_dem"
  Bus Creator/1 -> YaoKong_dem/1  "YaoKong"
  brake_emerg/1 -> Bus Creator/5  "brake_emerg"
  HAC/1 -> Bus Creator/6  "HAC"

== system DDCU_wxt_v02_forA/MainControl/mode_control ==
  mode_dem_out : Inport
  Signals : Inport  Port=2
  Multiport Switch : MultiPortSwitch  DataPortOrder=Zero-based contiguous  Inputs=6
  Park : Subsystem  TreatAsAtomicUnit=on
  Switch Case : SwitchCase  CaseConditions={0,1,2,3,4,5}  ShowDefaultCase=off
  backward : Subsystem  Commented=on  TreatAsAtomicUnit=on
  center_steer : Subsystem  TreatAsAtomicUnit=on
  emergency_stop : Subsystem  TreatAsAtomicUnit=on
  forward : Subsystem  TreatAsAtomicUnit=on
  neutral : Subsystem  TreatAsAtomicUnit=on
  com_dem : Outport
  wires:
  mode_dem_out/1 -> Multiport Switch/1, Switch Case/1
  Signals/1 -> emergency_stop/1(Signals), center_steer/1(Signals), backward/1(Signals), neutral/1(Signals), forward/1(Signals), Park/1(Signals)
  Switch Case/1 -> Park/Action
  Switch Case/6 -> emergency_stop/Action
  Switch Case/5 -> center_steer/Action
  Switch Case/4 -> backward/Action
  Switch Case/3 -> neutral/Action
  Switch Case/2 -> forward/Action
  Park/1(park_dem) -> Multiport Switch/2
  forward/1(forward_dem) -> Multiport Switch/3
  backward/1(backward_dem) -> Multiport Switch/5
  neutral/1(neutral_dem) -> Multiport Switch/4
  center_steer/1(center_steer_dem) -> Multiport Switch/6
  emergency_stop/1(emergency_stop_dem) -> Multiport Switch/7
  Multiport Switch/1 -> com_dem/1

== system DDCU_wxt_v02_forA/MainControl/mode_switch ==
  Signals : Inport
  Bus Selector : BusSelector  OutputSignals=YaoKong.mode_dem,YaoKong.brake_emerg,DriveMotor.speed_act_lf,DriveMotor.speed_act_lr,DriveMotor.speed_act_rf,DriveMotor.speed_act_rr,IMU.v_act
  Constant : Constant
  Constant1 : Constant  Value=v_thr_park
  Constant2 : Constant  Value=speed_thr_park
  Memory : Memory
  mode_switch : MATLAB Function  TreatAsAtomicUnit=on
  mode_dem_out : Outport
  wires:
  Memory/1 -> mode_switch/10(mode_dem_out_pre)
  Signals/1 -> Bus Selector/1
  Bus Selector/3 -> mode_switch/3(speed_act_lf)  "<speed_act_lf>"
  Bus Selector/2 -> mode_switch/2(brake_emerg)  "<brake_emerg>"
  Bus Selector/1 -> mode_switch/1(mode_dem)  "<mode_dem>"
  Bus Selector/5 -> mode_switch/5(speed_act_rf)  "<speed_act_rf>"
  Bus Selector/4 -> mode_switch/4(speed_act_lr)  "<speed_act_lr>"
  Bus Selector/6 -> mode_switch/6(speed_act_rr)  "<speed_act_rr>"
  Bus Selector/7 -> mode_switch/7(v_act)  "<v_act>"
  mode_switch/1(mode_dem_out) -> Memory/1
  Constant/1 -> mode_dem_out/1
  Constant2/1 -> mode_switch/9(speed_thr_park)
  Constant1/1 -> mode_switch/8(v_thr_park)

== system DDCU_wxt_v02_forA/OutputSignalProcess/VCU_ESC ==
  VVMS_BrkSts_flg_in : Inport
  VVMS_ParkSts_flg_in : Inport  Port=2
  VVMS_BrkPSetLe_MPa_in : Inport  Port=3
  VVMS_BrkPSetRi_MPa_in : Inport  Port=4
  Conv{1..8} (8 alike) : DataTypeConversion
  VCU_ESC_DLC : Constant  Value=8  OutDataTypeStr=uint8
  VCU_ESC_DLC_Out : Terminator
  VCU_ESC_ID : Constant  Value=2364992240  OutDataTypeStr=single
  VCU_ESC_ID_Out : Terminator
  VCU_ESC_mux : Mux  Inputs=8
  VVMS_BrkPSetLe_MPa : Subsystem
  VVMS_BrkPSetRi_MPa : Subsystem
  VVMS_BrkSts_flg : Subsystem
  VVMS_ParkSts_flg : Subsystem
  or{1..8} (8 alike) : simulink/Logic and Bit Operations/Bitwise Operator  logicop=OR  UseBitMask=off  NumInputPorts=4  BitMask=bin2dec('11011001')  BitMaskRealWorld=Stored Integer
  output : Outport
  wires:
  VCU_ESC_mux/1 -> output/1
  VVMS_BrkSts_flg/1(output1) -> or1/1
  VVMS_BrkSts_flg/2(output2) -> or2/1
  VVMS_BrkSts_flg/3(output3) -> or3/1
  VVMS_BrkSts_flg/4(output4) -> or4/1
  VVMS_BrkSts_flg/5(output5) -> or5/1
  VVMS_BrkSts_flg/6(output6) -> or6/1
  VVMS_BrkSts_flg/7(output7) -> or7/1
  VVMS_BrkSts_flg/8(output8) -> or8/1
  VVMS_ParkSts_flg/1(output1) -> or1/2
  VVMS_ParkSts_flg/2(output2) -> or2/2
  VVMS_ParkSts_flg/3(output3) -> or3/2
  VVMS_ParkSts_flg/4(output4) -> or4/2
  VVMS_ParkSts_flg/5(output5) -> or5/2
  VVMS_ParkSts_flg/6(output6) -> or6/2
  VVMS_ParkSts_flg/7(output7) -> or7/2
  VVMS_ParkSts_flg/8(output8) -> or8/2
  VVMS_BrkPSetRi_MPa/1(output1) -> or1/3
  VVMS_BrkPSetRi_MPa/2(output2) -> or2/3
  VVMS_BrkPSetRi_MPa/3(output3) -> or3/3
  VVMS_BrkPSetRi_MPa/4(output4) -> or4/3
  VVMS_BrkPSetRi_MPa/5(output5) -> or5/3
  VVMS_BrkPSetRi_MPa/6(output6) -> or6/3
  VVMS_BrkPSetRi_MPa/7(output7) -> or7/3
  VVMS_BrkPSetRi_MPa/8(output8) -> or8/3
  VVMS_BrkPSetLe_MPa/1(output1) -> or1/4
  VVMS_BrkPSetLe_MPa/2(output2) -> or2/4
  VVMS_BrkPSetLe_MPa/3(output3) -> or3/4
  VVMS_BrkPSetLe_MPa/4(output4) -> or4/4
  VVMS_BrkPSetLe_MPa/5(output5) -> or5/4
  VVMS_BrkPSetLe_MPa/6(output6) -> or6/4
  VVMS_BrkPSetLe_MPa/7(output7) -> or7/4
  VVMS_BrkPSetLe_MPa/8(output8) -> or8/4
  or1/1 -> Conv1/1
  Conv1/1 -> VCU_ESC_mux/1
  or2/1 -> Conv2/1
  Conv2/1 -> VCU_ESC_mux/2
  or3/1 -> Conv3/1
  Conv3/1 -> VCU_ESC_mux/3
  or4/1 -> Conv4/1
  Conv4/1 -> VCU_ESC_mux/4
  or5/1 -> Conv5/1
  Conv5/1 -> VCU_ESC_mux/5
  or6/1 -> Conv6/1
  Conv6/1 -> VCU_ESC_mux/6
  or7/1 -> Conv7/1
  Conv7/1 -> VCU_ESC_mux/7
  or8/1 -> Conv8/1
  Conv8/1 -> VCU_ESC_mux/8
  VCU_ESC_ID/1 -> VCU_ESC_ID_Out/1
  VCU_ESC_DLC/1 -> VCU_ESC_DLC_Out/1
  VVMS_BrkSts_flg_in/1 -> VVMS_BrkSts_flg/1(VVMS_BrkSts_flg)
  VVMS_ParkSts_flg_in/1 -> VVMS_ParkSts_flg/1(VVMS_ParkSts_flg)
  VVMS_BrkPSetRi_MPa_in/1 -> VVMS_BrkPSetRi_MPa/1(VVMS_BrkPSetRi_MPa)
  VVMS_BrkPSetLe_MPa_in/1 -> VVMS_BrkPSetLe_MPa/1(VVMS_BrkPSetLe_MPa)

== system DDCU_wxt_v02_forA/OutputSignalProcess/VCU_MCU1 ==
  M1Enable_in : Inport
  M1Mode_in : Inport  Port=2
  M1Drive_in : Inport  Port=3
  M1TorqueSet_in : Inport  Port=4
  M1SpeedLimit_in : Inport  Port=5
  M2Enable_in : Inport  Port=6
  M2Mode_in : Inport  Port=7
  M2Drive_in : Inport  Port=8
  M2TorqueSet_in : Inport  Port=9
  M2SpeedLimit_in : Inport  Port=10
  MCU1HeartBeat_in : Inport  Port=11
  Conv{1..8} (8 alike) : DataTypeConversion
  M1Drive : Subsystem
  M1Enable : Subsystem
  M1Mode : Subsystem
  M1SpeedLimit : Subsystem
  M1TorqueSet : Subsystem
  M2Drive : Subsystem
  M2Enable : Subsystem
  M2Mode : Subsystem
  M2SpeedLimit : Subsystem
  M2TorqueSet : Subsystem
  MCU1HeartBeat : Subsystem
  VCU_MCU1_DLC : Constant  Value=8  OutDataTypeStr=uint8
  VCU_MCU1_DLC_Out : Terminator
  VCU_MCU1_ID : Constant  Value=2348937217  OutDataTypeStr=single
  VCU_MCU1_ID_Out : Terminator
  VCU_MCU1_mux : Mux  Inputs=8
  or{1..8} (8 alike) : simulink/Logic and Bit Operations/Bitwise Operator  logicop=OR  UseBitMask=off  NumInputPorts=11  BitMask=bin2dec('11011001')  BitMaskRealWorld=Stored Integer
  output : Outport
  wires:
  VCU_MCU1_mux/1 -> output/1
  MCU1HeartBeat/1(output1) -> or1/1
  MCU1HeartBeat/2(output2) -> or2/1
  MCU1HeartBeat/3(output3) -> or3/1
  MCU1HeartBeat/4(output4) -> or4/1
  MCU1HeartBeat/5(output5) -> or5/1
  MCU1HeartBeat/6(output6) -> or6/1
  MCU1HeartBeat/7(output7) -> or7/1
  MCU1HeartBeat/8(output8) -> or8/1
  M2TorqueSet/1(output1) -> or1/2
  M2TorqueSet/2(output2) -> or2/2
  M2TorqueSet/3(output3) -> or3/2
  M2TorqueSet/4(output4) -> or4/2
  M2TorqueSet/5(output5) -> or5/2
  M2TorqueSet/6(output6) -> or6/2
  M2TorqueSet/7(output7) -> or7/2
  M2TorqueSet/8(output8) -> or8/2
  M2SpeedLimit/1(output1) -> or1/3
  M2SpeedLimit/2(output2) -> or2/3
  M2SpeedLimit/3(output3) -> or3/3
  M2SpeedLimit/4(output4) -> or4/3
  M2SpeedLimit/5(output5) -> or5/3
  M2SpeedLimit/6(output6) -> or6/3
  M2SpeedLimit/7(output7) -> or7/3
  M2SpeedLimit/8(output8) -> or8/3
  M2Mode/1(output1) -> or1/4
  M2Mode/2(output2) -> or2/4
  M2Mode/3(output3) -> or3/4
  M2Mode/4(output4) -> or4/4
  M2Mode/5(output5) -> or5/4
  M2Mode/6(output6) -> or6/4
  M2Mode/7(output7) -> or7/4
  M2Mode/8(output8) -> or8/4
  M2Enable/1(output1) -> or1/5
  M2Enable/2(output2) -> or2/5
  M2Enable/3(output3) -> or3/5
  M2Enable/4(output4) -> or4/5
  M2Enable/5(output5) -> or5/5
  M2Enable/6(output6) -> or6/5
  M2Enable/7(output7) -> or7/5
  M2Enable/8(output8) -> or8/5
  M2Drive/1(output1) -> or1/6
  M2Drive/2(output2) -> or2/6
  M2Drive/3(output3) -> or3/6
  M2Drive/4(output4) -> or4/6
  M2Drive/5(output5) -> or5/6
  M2Drive/6(output6) -> or6/6
  M2Drive/7(output7) -> or7/6
  M2Drive/8(output8) -> or8/6
  M1TorqueSet/1(output1) -> or1/7
  M1TorqueSet/2(output2) -> or2/7
  M1TorqueSet/3(output3) -> or3/7
  M1TorqueSet/4(output4) -> or4/7
  M1TorqueSet/5(output5) -> or5/7
  M1TorqueSet/6(output6) -> or6/7
  M1TorqueSet/7(output7) -> or7/7
  M1TorqueSet/8(output8) -> or8/7
  M1SpeedLimit/1(output1) -> or1/8
  M1SpeedLimit/2(output2) -> or2/8
  M1SpeedLimit/3(output3) -> or3/8
  M1SpeedLimit/4(output4) -> or4/8
  M1SpeedLimit/5(output5) -> or5/8
  M1SpeedLimit/6(output6) -> or6/8
  M1SpeedLimit/7(output7) -> or7/8
  M1SpeedLimit/8(output8) -> or8/8
  M1Mode/1(output1) -> or1/9
  M1Mode/2(output2) -> or2/9
  M1Mode/3(output3) -> or3/9
  M1Mode/4(output4) -> or4/9
  M1Mode/5(output5) -> or5/9
  M1Mode/6(output6) -> or6/9
  M1Mode/7(output7) -> or7/9
  M1Mode/8(output8) -> or8/9
  M1Enable/1(output1) -> or1/10
  M1Enable/2(output2) -> or2/10
  M1Enable/3(output3) -> or3/10
  M1Enable/4(output4) -> or4/10
  M1Enable/5(output5) -> or5/10
  M1Enable/6(output6) -> or6/10
  M1Enable/7(output7) -> or7/10
  M1Enable/8(output8) -> or8/10
  M1Drive/1(output1) -> or1/11
  M1Drive/2(output2) -> or2/11
  M1Drive/3(output3) -> or3/11
  M1Drive/4(output4) -> or4/11
  M1Drive/5(output5) -> or5/11
  M1Drive/6(output6) -> or6/11
  M1Drive/7(output7) -> or7/11
  M1Drive/8(output8) -> or8/11
  or1/1 -> Conv1/1
  Conv1/1 -> VCU_MCU1_mux/1
  or2/1 -> Conv2/1
  Conv2/1 -> VCU_MCU1_mux/2
  or3/1 -> Conv3/1
  Conv3/1 -> VCU_MCU1_mux/3
  or4/1 -> Conv4/1
  Conv4/1 -> VCU_MCU1_mux/4
  or5/1 -> Conv5/1
  Conv5/1 -> VCU_MCU1_mux/5
  or6/1 -> Conv6/1
  Conv6/1 -> VCU_MCU1_mux/6
  or7/1 -> Conv7/1
  Conv7/1 -> VCU_MCU1_mux/7
  or8/1 -> Conv8/1
  Conv8/1 -> VCU_MCU1_mux/8
  VCU_MCU1_ID/1 -> VCU_MCU1_ID_Out/1
  VCU_MCU1_DLC/1 -> VCU_MCU1_DLC_Out/1
  MCU1HeartBeat_in/1 -> MCU1HeartBeat/1(MCU1HeartBeat)
  M2TorqueSet_in/1 -> M2TorqueSet/1(M2TorqueSet)
  M2SpeedLimit_in/1 -> M2SpeedLimit/1(M2SpeedLimit)
  M2Mode_in/1 -> M2Mode/1(M2Mode)
  M2Enable_in/1 -> M2Enable/1(M2Enable)
  M2Drive_in/1 -> M2Drive/1(M2Drive)
  M1TorqueSet_in/1 -> M1TorqueSet/1(M1TorqueSet)
  M1SpeedLimit_in/1 -> M1SpeedLimit/1(M1SpeedLimit)
  M1Mode_in/1 -> M1Mode/1(M1Mode)
  M1Enable_in/1 -> M1Enable/1(M1Enable)
  M1Drive_in/1 -> M1Drive/1(M1Drive)

== system DDCU_wxt_v02_forA/OutputSignalProcess/VCU_MCU1_replace ==
  M2SpeedSet_in : Inport
  M1SpeedSet_in : Inport  Port=2
  MCU1HeartBeat_in : Inport  Port=3
  M2SpeedLimit_in : Inport  Port=4
  M2Mode_in : Inport  Port=5
  M2Enable_in : Inport  Port=6
  M2Drive_in : Inport  Port=7
  M1SpeedLimit_in : Inport  Port=8
  M1Mode_in : Inport  Port=9
  M1Enable_in : Inport  Port=10
  M1Drive_in : Inport  Port=11
  Conv{1..8} (8 alike) : DataTypeConversion
  M1Drive : Subsystem
  M1Enable : Subsystem
  M1Mode : Subsystem
  M1SpeedLimit : Subsystem
  M1SpeedSet : Subsystem
  M2Drive : Subsystem
  M2Enable : Subsystem
  M2Mode : Subsystem
  M2SpeedLimit : Subsystem
  M2SpeedSet : Subsystem
  MCU1HeartBeat : Subsystem
  VCU_MCU1_replace_DLC : Constant  Value=8  OutDataTypeStr=uint8
  VCU_MCU1_replace_DLC_Out : Terminator
  VCU_MCU1_replace_ID : Constant  Value=2348937233  OutDataTypeStr=single
  VCU_MCU1_replace_ID_Out : Terminator
  VCU_MCU1_replace_mux : Mux  Inputs=8
  or{1..8} (8 alike) : simulink/Logic and Bit Operations/Bitwise Operator  logicop=OR  UseBitMask=off  NumInputPorts=11  BitMask=bin2dec('11011001')  BitMaskRealWorld=Stored Integer
  output : Outport
  wires:
  VCU_MCU1_replace_mux/1 -> output/1
  M2SpeedSet/1(output1) -> or1/1
  M2SpeedSet/2(output2) -> or2/1
  M2SpeedSet/3(output3) -> or3/1
  M2SpeedSet/4(output4) -> or4/1
  M2SpeedSet/5(output5) -> or5/1
  M2SpeedSet/6(output6) -> or6/1
  M2SpeedSet/7(output7) -> or7/1
  M2SpeedSet/8(output8) -> or8/1
  M1SpeedSet/1(output1) -> or1/2
  M1SpeedSet/2(output2) -> or2/2
  M1SpeedSet/3(output3) -> or3/2
  M1SpeedSet/4(output4) -> or4/2
  M1SpeedSet/5(output5) -> or5/2
  M1SpeedSet/6(output6) -> or6/2
  M1SpeedSet/7(output7) -> or7/2
  M1SpeedSet/8(output8) -> or8/2
  MCU1HeartBeat/1(output1) -> or1/3
  MCU1HeartBeat/2(output2) -> or2/3
  MCU1HeartBeat/3(output3) -> or3/3
  MCU1HeartBeat/4(output4) -> or4/3
  MCU1HeartBeat/5(output5) -> or5/3
  MCU1HeartBeat/6(output6) -> or6/3
  MCU1HeartBeat/7(output7) -> or7/3
  MCU1HeartBeat/8(output8) -> or8/3
  M2SpeedLimit/1(output1) -> or1/4
  M2SpeedLimit/2(output2) -> or2/4
  M2SpeedLimit/3(output3) -> or3/4
  M2SpeedLimit/4(output4) -> or4/4
  M2SpeedLimit/5(output5) -> or5/4
  M2SpeedLimit/6(output6) -> or6/4
  M2SpeedLimit/7(output7) -> or7/4
  M2SpeedLimit/8(output8) -> or8/4
  M2Mode/1(output1) -> or1/5
  M2Mode/2(output2) -> or2/5
  M2Mode/3(output3) -> or3/5
  M2Mode/4(output4) -> or4/5
  M2Mode/5(output5) -> or5/5
  M2Mode/6(output6) -> or6/5
  M2Mode/7(output7) -> or7/5
  M2Mode/8(output8) -> or8/5
  M2Enable/1(output1) -> or1/6
  M2Enable/2(output2) -> or2/6
  M2Enable/3(output3) -> or3/6
  M2Enable/4(output4) -> or4/6
  M2Enable/5(output5) -> or5/6
  M2Enable/6(output6) -> or6/6
  M2Enable/7(output7) -> or7/6
  M2Enable/8(output8) -> or8/6
  M2Drive/1(output1) -> or1/7
  M2Drive/2(output2) -> or2/7
  M2Drive/3(output3) -> or3/7
  M2Drive/4(output4) -> or4/7
  M2Drive/5(output5) -> or5/7
  M2Drive/6(output6) -> or6/7
  M2Drive/7(output7) -> or7/7
  M2Drive/8(output8) -> or8/7
  M1SpeedLimit/1(output1) -> or1/8
  M1SpeedLimit/2(output2) -> or2/8
  M1SpeedLimit/3(output3) -> or3/8
  M1SpeedLimit/4(output4) -> or4/8
  M1SpeedLimit/5(output5) -> or5/8
  M1SpeedLimit/6(output6) -> or6/8
  M1SpeedLimit/7(output7) -> or7/8
  M1SpeedLimit/8(output8) -> or8/8
  M1Mode/1(output1) -> or1/9
  M1Mode/2(output2) -> or2/9
  M1Mode/3(output3) -> or3/9
  M1Mode/4(output4) -> or4/9
  M1Mode/5(output5) -> or5/9
  M1Mode/6(output6) -> or6/9
  M1Mode/7(output7) -> or7/9
  M1Mode/8(output8) -> or8/9
  M1Enable/1(output1) -> or1/10
  M1Enable/2(output2) -> or2/10
  M1Enable/3(output3) -> or3/10
  M1Enable/4(output4) -> or4/10
  M1Enable/5(output5) -> or5/10
  M1Enable/6(output6) -> or6/10
  M1Enable/7(output7) -> or7/10
  M1Enable/8(output8) -> or8/10
  M1Drive/1(output1) -> or1/11
  M1Drive/2(output2) -> or2/11
  M1Drive/3(output3) -> or3/11
  M1Drive/4(output4) -> or4/11
  M1Drive/5(output5) -> or5/11
  M1Drive/6(output6) -> or6/11
  M1Drive/7(output7) -> or7/11
  M1Drive/8(output8) -> or8/11
  or1/1 -> Conv1/1
  Conv1/1 -> VCU_MCU1_replace_mux/1
  or2/1 -> Conv2/1
  Conv2/1 -> VCU_MCU1_replace_mux/2
  or3/1 -> Conv3/1
  Conv3/1 -> VCU_MCU1_replace_mux/3
  or4/1 -> Conv4/1
  Conv4/1 -> VCU_MCU1_replace_mux/4
  or5/1 -> Conv5/1
  Conv5/1 -> VCU_MCU1_replace_mux/5
  or6/1 -> Conv6/1
  Conv6/1 -> VCU_MCU1_replace_mux/6
  or7/1 -> Conv7/1
  Conv7/1 -> VCU_MCU1_replace_mux/7
  or8/1 -> Conv8/1
  Conv8/1 -> VCU_MCU1_replace_mux/8
  VCU_MCU1_replace_ID/1 -> VCU_MCU1_replace_ID_Out/1
  VCU_MCU1_replace_DLC/1 -> VCU_MCU1_replace_DLC_Out/1
  M2SpeedSet_in/1 -> M2SpeedSet/1(M2SpeedSet)
  M1SpeedSet_in/1 -> M1SpeedSet/1(M1SpeedSet)
  MCU1HeartBeat_in/1 -> MCU1HeartBeat/1(MCU1HeartBeat)
  M2SpeedLimit_in/1 -> M2SpeedLimit/1(M2SpeedLimit)
  M2Mode_in/1 -> M2Mode/1(M2Mode)
  M2Enable_in/1 -> M2Enable/1(M2Enable)
  M2Drive_in/1 -> M2Drive/1(M2Drive)
  M1SpeedLimit_in/1 -> M1SpeedLimit/1(M1SpeedLimit)
  M1Mode_in/1 -> M1Mode/1(M1Mode)
  M1Enable_in/1 -> M1Enable/1(M1Enable)
  M1Drive_in/1 -> M1Drive/1(M1Drive)

== system DDCU_wxt_v02_forA/OutputSignalProcess/VCU_MCU2 ==
  M3Enable_in : Inport
  M3Mode_in : Inport  Port=2
  M3Drive_in : Inport  Port=3
  M3TorqueSet_in : Inport  Port=4
  M3SpeedLimit_in : Inport  Port=5
  M4Enable_in : Inport  Port=6
  M4Mode_in : Inport  Port=7
  M4Drive_in : Inport  Port=8
  M4TorqueSet_in : Inport  Port=9
  M4SpeedLimit_in : Inport  Port=10
  MCU2HeartBeat_in : Inport  Port=11
  Conv{1..8} (8 alike) : DataTypeConversion
  M3Drive : Subsystem
  M3Enable : Subsystem
  M3Mode : Subsystem
  M3SpeedLimit : Subsystem
  M3TorqueSet : Subsystem
  M4Drive : Subsystem
  M4Enable : Subsystem
  M4Mode : Subsystem
  M4SpeedLimit : Subsystem
  M4TorqueSet : Subsystem
  MCU2HeartBeat : Subsystem
  VCU_MCU2_DLC : Constant  Value=8  OutDataTypeStr=uint8
  VCU_MCU2_DLC_Out : Terminator
  VCU_MCU2_ID : Constant  Value=2348937218  OutDataTypeStr=single
  VCU_MCU2_ID_Out : Terminator
  VCU_MCU2_mux : Mux  Inputs=8
  or{1..8} (8 alike) : simulink/Logic and Bit Operations/Bitwise Operator  logicop=OR  UseBitMask=off  NumInputPorts=11  BitMask=bin2dec('11011001')  BitMaskRealWorld=Stored Integer
  output : Outport
  wires:
  VCU_MCU2_mux/1 -> output/1
  MCU2HeartBeat/1(output1) -> or1/1
  MCU2HeartBeat/2(output2) -> or2/1
  MCU2HeartBeat/3(output3) -> or3/1
  MCU2HeartBeat/4(output4) -> or4/1
  MCU2HeartBeat/5(output5) -> or5/1
  MCU2HeartBeat/6(output6) -> or6/1
  MCU2HeartBeat/7(output7) -> or7/1
  MCU2HeartBeat/8(output8) -> or8/1
  M4TorqueSet/1(output1) -> or1/2
  M4TorqueSet/2(output2) -> or2/2
  M4TorqueSet/3(output3) -> or3/2
  M4TorqueSet/4(output4) -> or4/2
  M4TorqueSet/5(output5) -> or5/2
  M4TorqueSet/6(output6) -> or6/2
  M4TorqueSet/7(output7) -> or7/2
  M4TorqueSet/8(output8) -> or8/2
  M4SpeedLimit/1(output1) -> or1/3
  M4SpeedLimit/2(output2) -> or2/3
  M4SpeedLimit/3(output3) -> or3/3
  M4SpeedLimit/4(output4) -> or4/3
  M4SpeedLimit/5(output5) -> or5/3
  M4SpeedLimit/6(output6) -> or6/3
  M4SpeedLimit/7(output7) -> or7/3
  M4SpeedLimit/8(output8) -> or8/3
  M4Mode/1(output1) -> or1/4
  M4Mode/2(output2) -> or2/4
  M4Mode/3(output3) -> or3/4
  M4Mode/4(output4) -> or4/4
  M4Mode/5(output5) -> or5/4
  M4Mode/6(output6) -> or6/4
  M4Mode/7(output7) -> or7/4
  M4Mode/8(output8) -> or8/4
  M4Enable/1(output1) -> or1/5
  M4Enable/2(output2) -> or2/5
  M4Enable/3(output3) -> or3/5
  M4Enable/4(output4) -> or4/5
  M4Enable/5(output5) -> or5/5
  M4Enable/6(output6) -> or6/5
  M4Enable/7(output7) -> or7/5
  M4Enable/8(output8) -> or8/5
  M4Drive/1(output1) -> or1/6
  M4Drive/2(output2) -> or2/6
  M4Drive/3(output3) -> or3/6
  M4Drive/4(output4) -> or4/6
  M4Drive/5(output5) -> or5/6
  M4Drive/6(output6) -> or6/6
  M4Drive/7(output7) -> or7/6
  M4Drive/8(output8) -> or8/6
  M3TorqueSet/1(output1) -> or1/7
  M3TorqueSet/2(output2) -> or2/7
  M3TorqueSet/3(output3) -> or3/7
  M3TorqueSet/4(output4) -> or4/7
  M3TorqueSet/5(output5) -> or5/7
  M3TorqueSet/6(output6) -> or6/7
  M3TorqueSet/7(output7) -> or7/7
  M3TorqueSet/8(output8) -> or8/7
  M3SpeedLimit/1(output1) -> or1/8
  M3SpeedLimit/2(output2) -> or2/8
  M3SpeedLimit/3(output3) -> or3/8
  M3SpeedLimit/4(output4) -> or4/8
  M3SpeedLimit/5(output5) -> or5/8
  M3SpeedLimit/6(output6) -> or6/8
  M3SpeedLimit/7(output7) -> or7/8
  M3SpeedLimit/8(output8) -> or8/8
  M3Mode/1(output1) -> or1/9
  M3Mode/2(output2) -> or2/9
  M3Mode/3(output3) -> or3/9
  M3Mode/4(output4) -> or4/9
  M3Mode/5(output5) -> or5/9
  M3Mode/6(output6) -> or6/9
  M3Mode/7(output7) -> or7/9
  M3Mode/8(output8) -> or8/9
  M3Enable/1(output1) -> or1/10
  M3Enable/2(output2) -> or2/10
  M3Enable/3(output3) -> or3/10
  M3Enable/4(output4) -> or4/10
  M3Enable/5(output5) -> or5/10
  M3Enable/6(output6) -> or6/10
  M3Enable/7(output7) -> or7/10
  M3Enable/8(output8) -> or8/10
  M3Drive/1(output1) -> or1/11
  M3Drive/2(output2) -> or2/11
  M3Drive/3(output3) -> or3/11
  M3Drive/4(output4) -> or4/11
  M3Drive/5(output5) -> or5/11
  M3Drive/6(output6) -> or6/11
  M3Drive/7(output7) -> or7/11
  M3Drive/8(output8) -> or8/11
  or1/1 -> Conv1/1
  Conv1/1 -> VCU_MCU2_mux/1
  or2/1 -> Conv2/1
  Conv2/1 -> VCU_MCU2_mux/2
  or3/1 -> Conv3/1
  Conv3/1 -> VCU_MCU2_mux/3
  or4/1 -> Conv4/1
  Conv4/1 -> VCU_MCU2_mux/4
  or5/1 -> Conv5/1
  Conv5/1 -> VCU_MCU2_mux/5
  or6/1 -> Conv6/1
  Conv6/1 -> VCU_MCU2_mux/6
  or7/1 -> Conv7/1
  Conv7/1 -> VCU_MCU2_mux/7
  or8/1 -> Conv8/1
  Conv8/1 -> VCU_MCU2_mux/8
  VCU_MCU2_ID/1 -> VCU_MCU2_ID_Out/1
  VCU_MCU2_DLC/1 -> VCU_MCU2_DLC_Out/1
  MCU2HeartBeat_in/1 -> MCU2HeartBeat/1(MCU2HeartBeat)
  M4TorqueSet_in/1 -> M4TorqueSet/1(M4TorqueSet)
  M4SpeedLimit_in/1 -> M4SpeedLimit/1(M4SpeedLimit)
  M4Mode_in/1 -> M4Mode/1(M4Mode)
  M4Enable_in/1 -> M4Enable/1(M4Enable)
  M4Drive_in/1 -> M4Drive/1(M4Drive)
  M3TorqueSet_in/1 -> M3TorqueSet/1(M3TorqueSet)
  M3SpeedLimit_in/1 -> M3SpeedLimit/1(M3SpeedLimit)
  M3Mode_in/1 -> M3Mode/1(M3Mode)
  M3Enable_in/1 -> M3Enable/1(M3Enable)
  M3Drive_in/1 -> M3Drive/1(M3Drive)

== matlab function DDCU_wxt_v02_forA/MainControl/mode_control/forward/forward/Brake/HeartBeat ==
  data: life_pre input; life output
function life = fcn(life_pre)
%#codegen
life=life_pre+1;
if life>15
    life=0;
end
end

== matlab function DDCU_wxt_v02_forA/MainControl/mode_control/forward/forward/Brake/HeartBeat1 ==
  data: life_pre input; life output
function life = fcn(life_pre)
%#codegen
life=life_pre+1;
if life>15
    life=0;
end
end

== matlab function DDCU_wxt_v02_forA/MainControl/mode_control/neutral/neutral/HeartBeat1 ==
  data: life_pre input; life output
function life = fcn(life_pre)
%#codegen
life=life_pre+1;
if life>15
    life=0;
end
end
